simulink model "Regulateur_Proportionel_Integrale_Tuning"  (R2017a)
settings: Solver=VariableStepAuto  StartTime=0.0  StopTime=10  RelTol=1e-3
libraries: simulink x1
settings Model: Creator=PC  LastModifiedBy=PC

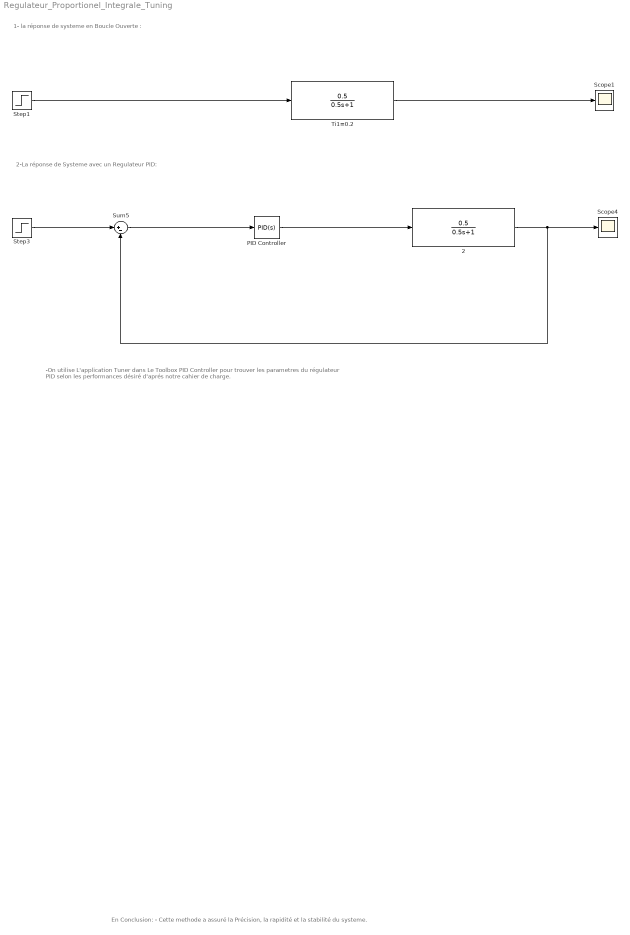
== system Regulateur_Proportionel_Integrale_Tuning ==
  note: -On utilise L'application Tuner dans Le Toolbox PID Controller pour trouver les parametres du régulateur PID selon les performances désiré d'aprés notre cahier de charge.
  note: En Conclusion:
      | - Cette methode a assuré la Précision, la rapidité et la stabilité du systeme.
  note: 1- la réponse de systeme en Boucle Ouverte :
  note: 2-La réponse de Systeme avec un Regulateur PID:
  2 : TransferFcn  Numerator=[0.5]  Denominator=[0.5 1]
  PID Controller : simulink/Continuous/PID Controller  Controller=PID  TimeDomain=Continuous-time  SampleTime=-1  IntegratorMethod=Forward Euler  FilterMethod=Forward Euler  Form=Parallel  UseFilter=on  ControllerParametersSource=internal  P=3.15643022892188  I=8.19535230540206  D=0.0919867808867041  N=5.85245289208397  InitialConditionSource=internal  InitialConditionForIntegrator=0  InitialConditionForFilter=0  ExternalReset=none  LimitOutput=off  UpperSaturationLimit=inf  LowerSaturationLimit=-inf  LinearizeAsGain=on  AntiWindupMode=none  Kb=1  TrackingMode=off  Kt=1  PParamMin=[]  PParamMax=[]  IParamMin=[]  IParamMax=[]  DParamMin=[]  DParamMax=[]  NParamMin=[]  NParamMax=[]  KbParamMin=[]  KbParamMax=[]  KtParamMin=[]  KtParamMax=[]  POutMin=[]  POutMax=[]  IOutMin=[]  IOutMax=[]  DOutMin=[]  DOutMax=[]  NOutMin=[]  NOutMax=[]  KbOutMin=[]  KbOutMax=[]  KtOutMin=[]  KtOutMax=[]  IntegratorOutMin=[]  IntegratorOutMax=[]  FilterOutMin=[]  FilterOutMax=[]  SumOutMin=[]  SumOutMax=[]  SumI1OutMin=[]  SumI1OutMax=[]  SumI2OutMin=[]  SumI2OutMax=[]  SumI3OutMin=[]  SumI3OutMax=[]  SumDOutMin=[]  SumDOutMax=[]  SaturationOutMin=[]  SaturationOutMax=[]  IntegratorContinuousStateAttributes=''  IntegratorStateMustResolveToSignalObject=off  IntegratorRTWStateStorageClass=Auto  FilterContinuousStateAttributes=''  FilterStateMustResolveToSignalObject=off  FilterRTWStateStorageClass=Auto  DifferentiatorICPrevScaledInput=0  DifferentiatorOutMin=[]  DifferentiatorOutMax=[]  InitialConditionSetting=State (most efficient)
  Scope1 : Scope
  Scope4 : Scope
  Step1 : Step  Time=0  SampleTime=0
  Step3 : Step  Time=0  SampleTime=0
  Sum5 : Sum  Inputs=|+-
  Ti1=0.2 : TransferFcn  Numerator=[0.5]  Denominator=[0.5 1]
  wires:
  Ti1=0.2/1 -> Scope1/1
  Step1/1 -> Ti1=0.2/1
  2/1 -> Scope4/1, Sum5/2
  Step3/1 -> Sum5/1
  Sum5/1 -> PID Controller/1
  PID Controller/1 -> 2/1
